simulink model "mechPower"  (R2014a)
settings: Solver=ode45  StartTime=0.0  StopTime=10.0  RelTol=1e-3
undefined symbols (not defined in the file or in its folder): dumping, H, Wn, ws
settings Model: Creator=Grid  LastModifiedBy=Grid

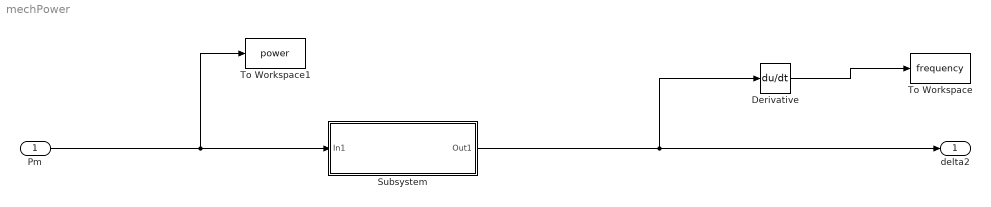
== system mechPower ==
  Pm : Inport
  Derivative : Derivative
  Subsystem : Subsystem
  To Workspace : ToWorkspace  VariableName=frequency  SaveFormat=Structure With Time  SampleTime=-1
  To Workspace1 : ToWorkspace  VariableName=power  SaveFormat=Structure With Time  SampleTime=-1
  delta2 : Outport  RequirementInfo={'linktype_rmi_matlab' 'Diesel' '@736250.2' 'true' 'mechPower' '' } %GIDa_5873d39b_2e25_4704_894b_5b50887017fb
  wires:
  Pm/1 -> To Workspace1/1, Subsystem/1(In1)
  Subsystem/1(Out1) -> Derivative/1, delta2/1
  Derivative/1 -> To Workspace/1

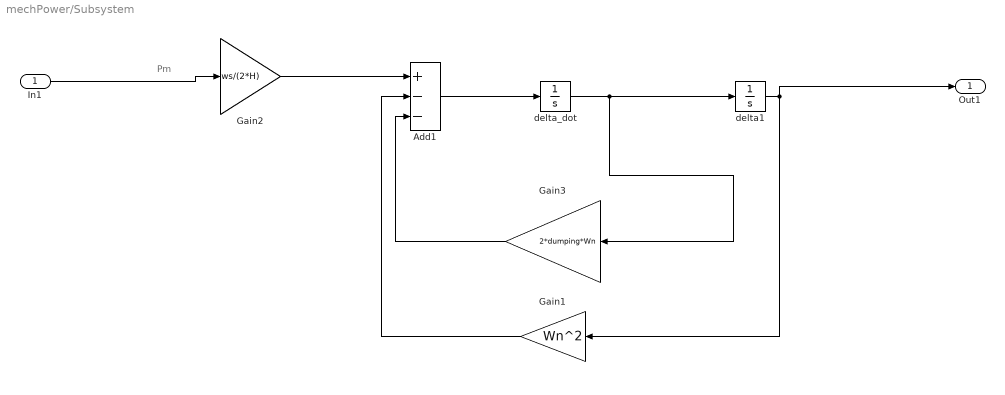
== system mechPower/Subsystem ==
  note: Pm
  In1 : Inport
  Add1 : Sum  Inputs=+--
  Gain1 : Gain  Gain=Wn^2
  Gain2 : Gain  Gain=ws/(2*H)
  Gain3 : Gain  Gain=2*dumping*Wn
  "delta1 " : Integrator
  delta_dot : Integrator
  Out1 : Outport
  wires:
  Gain1/1 -> Add1/2
  Add1/1 -> delta_dot/1
  delta_dot/1 -> Gain3/1, "delta1 "/1
  Gain2/1 -> Add1/1
  Gain3/1 -> Add1/3
  In1/1 -> Gain2/1
  "delta1 "/1 -> Out1/1, Gain1/1
